simulink model "PreliminaryRippleTest"  (R2024a)
settings: Solver=VariableStepAuto  StartTime=0.0  StopTime=0.05  MaxStep=1e-6  RelTol=1e-3
libraries: cstblocks x4
settings Model: Creator=FactCore  LastModifiedBy=FactCore

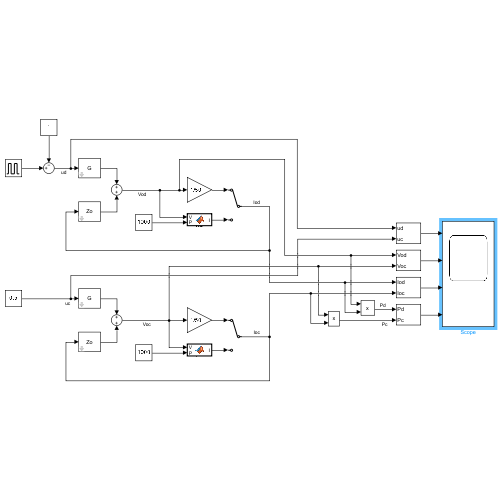
[thumbnail: Simulink's stored preview of the top-level diagram]
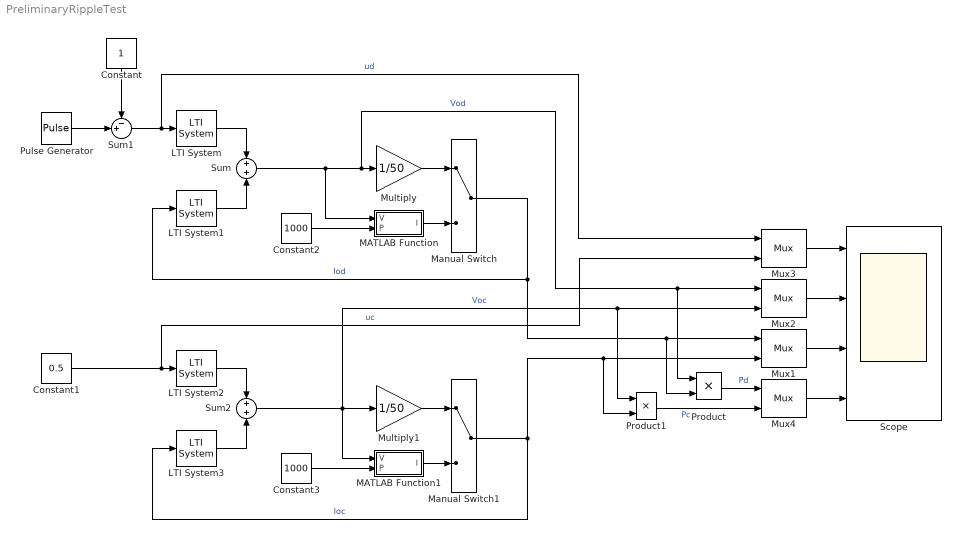
== system PreliminaryRippleTest ==
  Constant : Constant
  Constant1 : Constant  Value=0.5
  Constant2 : Constant  Value=1000
  Constant3 : Constant  Value=1000
  LTI System : cstblocks/LTI System  sys=G  IC=[]  PadeOrder=0
  LTI System1 : cstblocks/LTI System  sys=Zo  IC=[]  PadeOrder=0
  LTI System2 : cstblocks/LTI System  sys=G  IC=[]  PadeOrder=0
  LTI System3 : cstblocks/LTI System  sys=Zo  IC=[]  PadeOrder=0
  MATLAB Function : MATLAB Function  TreatAsAtomicUnit=on
  MATLAB Function1 : MATLAB Function  TreatAsAtomicUnit=on
  Manual Switch : ManualSwitch
  Manual Switch1 : ManualSwitch
  Multiply : Gain  Gain=1/50
  Multiply1 : Gain  Gain=1/50
  Mux{1..4} (4 alike) : Mux  Inputs=2
      settings: DisplayOption=signals
  Product : Product
  Product1 : Product
  Pulse Generator : DiscretePulseGenerator  PulseType=Time based  Amplitude=2  Period=100e-5  PulseWidth=75
  Scope : Scope  NumInputPorts=4
  Sum : Sum
  Sum1 : Sum  Inputs=-+|
  Sum2 : Sum
  wires:
  LTI System/1 -> Sum/1
  LTI System1/1 -> Sum/2
  Sum/1 -> Product/1, Mux2/1, Multiply/1, MATLAB Function/1(V)  "Vod"
  Manual Switch/1 -> Product/2, Mux1/1, LTI System1/1  "Iod"
  Pulse Generator/1 -> Sum1/2
  Sum1/1 -> Mux3/1, LTI System/1  "ud"
  Constant/1 -> Sum1/1
  Multiply/1 -> Manual Switch/1
  MATLAB Function/1(I) -> Manual Switch/2
  Constant2/1 -> MATLAB Function/2(P)
  Constant3/1 -> MATLAB Function1/2(P)
  MATLAB Function1/1(I) -> Manual Switch1/2
  Multiply1/1 -> Manual Switch1/1
  Constant1/1 -> Mux3/2, LTI System2/1  "uc"
  Manual Switch1/1 -> Product1/2, Mux1/2, LTI System3/1  "Ioc"
  Sum2/1 -> MATLAB Function1/1(V), Product1/1, Mux2/2, Multiply1/1  "Voc"
  LTI System3/1 -> Sum2/2
  LTI System2/1 -> Sum2/1
  Mux3/1 -> Scope/1
  Mux1/1 -> Scope/3
  Mux2/1 -> Scope/2
  Mux4/1 -> Scope/4
  Product1/1 -> Mux4/2  "Pc"
  Product/1 -> Mux4/1  "Pd"

== matlab function PreliminaryRippleTest/MATLAB Function ==
  data: V input; I output; P input
function I = fcn(V, P)

if V < 20
    I = 0;
    return
end

I = P/V;

== matlab function PreliminaryRippleTest/MATLAB Function1 ==
  data: V input; I output; P input
function I = fcn(V, P)

if V < 20
    I = 0;
    return
end

I = P/V;
